simulink model "second_proble"  (R2018a)
settings: Solver=VariableStepAuto  StartTime=0.0  StopTime=50  RelTol=1e-3
settings Model: Creator=lenovo  LastModifiedBy=lenovo

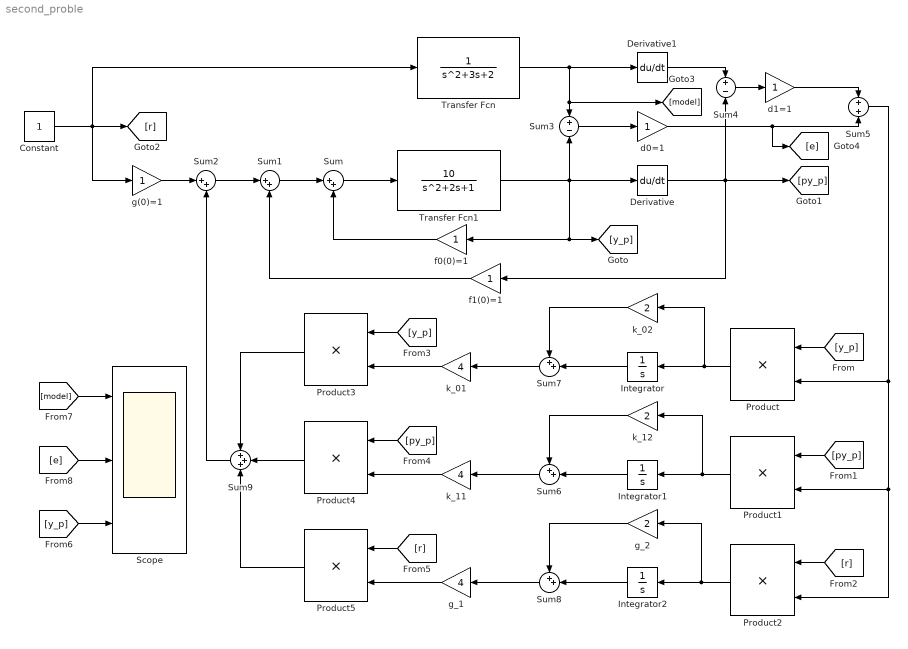
== system second_proble ==
  Constant : Constant
  Derivative : Derivative
  Derivative1 : Derivative
  Integrator : Integrator
  Integrator1 : Integrator
  Integrator2 : Integrator
  Product{,1..5} (6 alike) : Product
  Scope : Scope  NumInputPorts=3
  Sum : Sum  Inputs=|++
  Sum1 : Sum  Inputs=|++
  Sum2 : Sum  Inputs=|++
  Sum3 : Sum  Inputs=+|-
  Sum4 : Sum  Inputs=+|-
  Sum5 : Sum  Inputs=+|+
  Sum6 : Sum  Inputs=++|
  Sum7 : Sum  Inputs=++|
  Sum8 : Sum  Inputs=++|
  Sum9 : Sum  Inputs=+++
  Transfer Fcn : TransferFcn  Denominator=[1 3 2]
  Transfer Fcn1 : TransferFcn  Numerator=[10]
  d0=1 : Gain
  d1=1 : Gain
  f0(0)=1 : Gain
  f1(0)=1 : Gain
  g(0)=1 : Gain
  g_1 : Gain  Gain=4
  g_2 : Gain  Gain=2
  k_01 : Gain  Gain=4
  k_02 : Gain  Gain=2
  k_11 : Gain  Gain=4
  k_12 : Gain  Gain=2
  wires:
  Constant/1 -> Transfer Fcn/1, [r], g(0)=1/1
  Sum1/1 -> Sum/1
  Sum2/1 -> Sum1/1
  Sum/1 -> Transfer Fcn1/1
  Transfer Fcn/1 -> [model], Sum3/1, Derivative1/1
  Transfer Fcn1/1 -> Sum3/2, [y_p], f0(0)=1/1, Derivative/1
  Derivative/1 -> Sum4/2, [py_p], f1(0)=1/1
  Derivative1/1 -> Sum4/1
  Sum4/1 -> d1=1/1
  Sum3/1 -> d0=1/1
  d1=1/1 -> Sum5/1
  d0=1/1 -> [e], Sum5/2
  g(0)=1/1 -> Sum2/1
  f0(0)=1/1 -> Sum/2
  f1(0)=1/1 -> Sum1/2
  [y_p] -> Product/1
  [py_p] -> Product1/1
  [r] -> Product2/1
  Sum5/1 -> Product2/2, Product1/2, Product/2
  Product/1 -> k_02/1, Integrator/1
  Product1/1 -> k_12/1, Integrator1/1
  Product2/1 -> g_2/1, Integrator2/1
  k_02/1 -> Sum7/1
  Integrator/1 -> Sum7/2
  k_12/1 -> Sum6/1
  Integrator1/1 -> Sum6/2
  g_2/1 -> Sum8/1
  Integrator2/1 -> Sum8/2
  Sum7/1 -> k_01/1
  Sum6/1 -> k_11/1
  Sum8/1 -> g_1/1
  k_01/1 -> Product3/2
  k_11/1 -> Product4/2
  g_1/1 -> Product5/2
  [y_p] -> Product3/1
  [py_p] -> Product4/1
  [r] -> Product5/1
  Sum9/1 -> Sum2/2
  Product5/1 -> Sum9/3
  Product4/1 -> Sum9/2
  Product3/1 -> Sum9/1
  [y_p] -> Scope/3
  [model] -> Scope/1
  [e] -> Scope/2
